simulink model "LinearisedLQRPosition"  (R2024a)
settings: Solver=VariableStepAuto  StartTime=0.0  StopTime=10  RelTol=1e-3
undefined symbols (not defined in the file): A_pos, B_pos, C_pos, lqrd, Qpsi_pos, Qx_pos, Qy_pos, Qz_pos, Ts, Vehicle
libraries: simulink x1
settings Model: Creator=advay  LastModifiedBy=advay

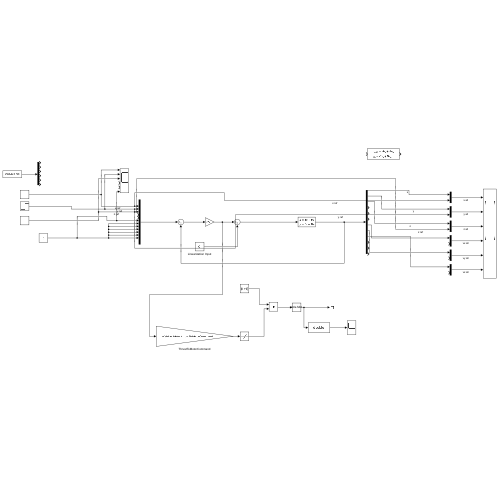
[thumbnail: Simulink's stored preview of the top-level diagram]
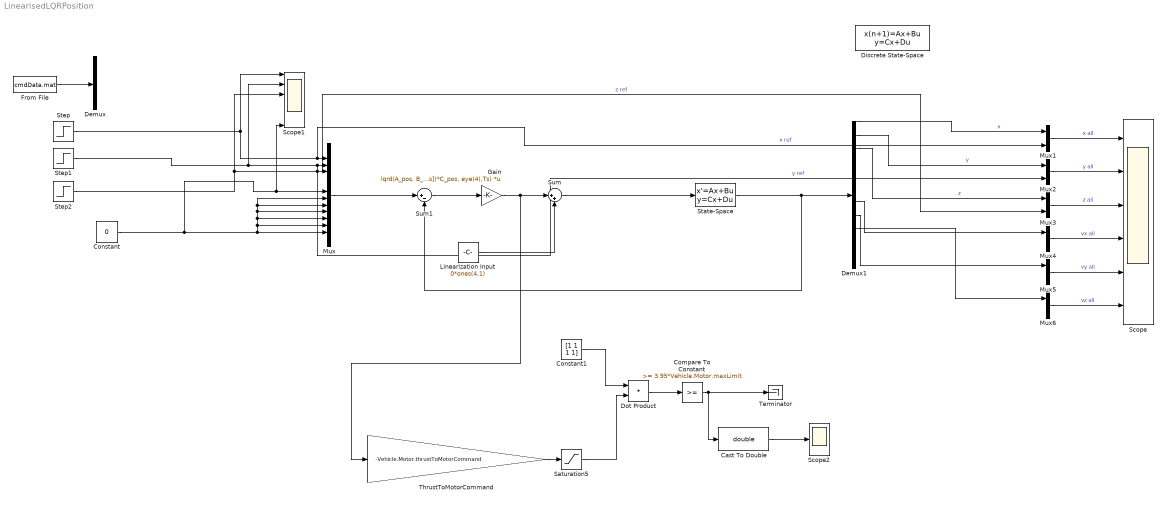
== system LinearisedLQRPosition ==
  Cast To Double : DataTypeConversion  OutDataTypeStr=double  SaturateOnIntegerOverflow=off  RndMeth=Floor
  Compare To Constant : simulink/Logic and Bit Operations/Compare To Constant  relop=>=  const=3.95*Vehicle.Motor.maxLimit  OutDataTypeStr=boolean
  Constant : Constant  Value=0  SampleTime=Ts
  Constant1 : Constant  Value=[1 1 1 1]  OutDataTypeStr=double
  Demux : Demux  Outputs=6
  Demux1 : Demux  Outputs=12
  Discrete State-Space : DiscreteStateSpace  A=A_pos  B=B_pos  C=eye(12)  D=zeros(12,4)  SampleTime=Ts
  Dot Product : DotProduct  OutDataTypeStr=Inherit: Inherit via internal rule
  From File : FromFile  FileName=cmdData.mat  SampleTime=Ts
  Gain : Gain  Gain=lqrd(A_pos, B_pos, C_pos'*diag([Qx_pos, Qy_pos, Qz_pos, Qpsi_pos])*C_pos, eye(4),Ts)  Multiplication=Matrix(K*u)
  Linearization Input : Constant  Value=0*ones(4,1)  OutDataTypeStr=double  SampleTime=Ts
  Mux : Mux  Inputs=12
  Mux{1..6} (6 alike) : Mux  Inputs=2
  Saturation5 : Saturate  UpperLimit=Vehicle.Motor.maxLimit  LowerLimit=Vehicle.Motor.minLimit
  Scope : Scope  NumInputPorts=6
  Scope1 : Scope  NumInputPorts=6
  Scope2 : Scope
  State-Space : StateSpace  A=A_pos  B=B_pos  C=eye(12)  D=zeros(12,4)  InitialCondition=0
  Step : Step  SampleTime=Ts
  Step1 : Step  Time=2  SampleTime=Ts
  Step2 : Step  Time=3  SampleTime=Ts
  Sum : Sum  Inputs=|++
  Sum1 : Sum  Inputs=|+-
  Terminator : Terminator
  ThrustToMotorCommand : Gain  Gain=-Vehicle.Motor.thrustToMotorCommand
  wires:
  Linearization Input/1 -> Sum/2
  Sum/1 -> State-Space/1
  State-Space/1 -> Sum1/2, Demux1/1
  Sum1/1 -> Gain/1
  Mux/1 -> Sum1/1
  Step/1 -> Mux1/2, Mux/1, Scope1/1  "x ref"
  Step1/1 -> Scope1/2, Mux2/2, Mux/2  "y ref"
  Step2/1 -> Scope1/3, Mux3/2, Mux/3  "z ref"
  Mux1/1 -> Scope/1  "x all"
  Mux2/1 -> Scope/2  "y all"
  Mux3/1 -> Scope/3  "z all"
  Mux4/1 -> Scope/4  "vx all"
  Mux5/1 -> Scope/5  "vy all"
  Mux6/1 -> Scope/6  "vz all"
  Demux1/1 -> Mux1/1  "x"
  Demux1/2 -> Mux2/1  "y"
  Demux1/3 -> Mux3/1  "z"
  Constant/1 -> Scope1/6, Mux/6, Mux/12, Mux/11, Mux/10, Mux/9, Mux/8, Mux/7
  Demux1/7 -> Mux4/1
  Demux1/8 -> Mux5/1
  Demux1/9 -> Mux6/1
  From File/1 -> Demux/1
  Gain/1 -> ThrustToMotorCommand/1, Sum/1
  Dot Product/1 -> Compare To Constant/1
  Saturation5/1 -> Dot Product/2
  Constant1/1 -> Dot Product/1
  ThrustToMotorCommand/1 -> Saturation5/1
  Compare To Constant/1 -> Cast To Double/1, Terminator/1
  Cast To Double/1 -> Scope2/1
